simulink model "blocks1"  (R2025a)
settings: Solver=VariableStepAuto  StartTime=0.0  StopTime=10.0  RelTol=1e-3
undefined symbols (not defined in the file or in its folder): physconst
libraries: phaseddetectlib x2, phasedstaplib x1
settings Model: Creator=Admin  LastModifiedBy=Admin

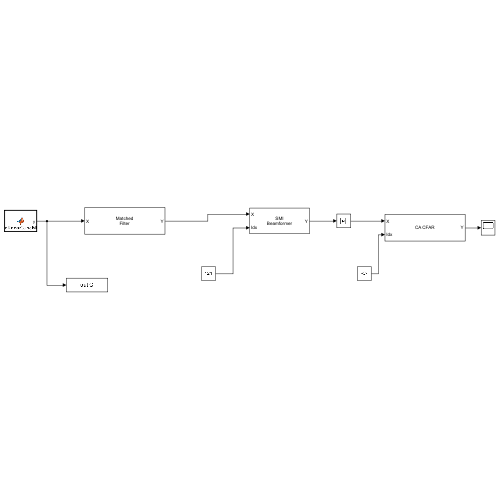
[thumbnail: Simulink's stored preview of the top-level diagram]
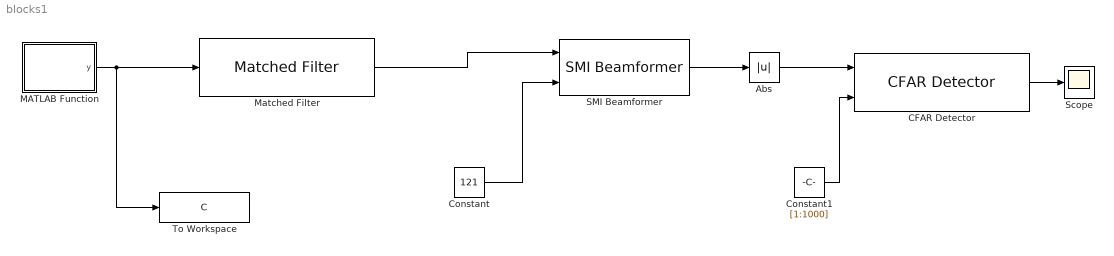
== system blocks1 ==
  Abs : Abs  SaturateOnIntegerOverflow=off
  CFAR Detector : phaseddetectlib/CFAR Detector  Method=CA  Rank=1  NumGuardCells=2  NumTrainingCells=2  ThresholdFactor=Auto  ProbabilityFalseAlarm=0.1  CustomThresholdFactor=1  OutputFormat=CUT result  ThresholdOutputPort=off  NoisePowerOutputPort=off  NumDetectionsSource=Auto  NumDetections=1  SimulateUsing=Interpreted execution
  Constant : Constant  Value=121
  Constant1 : Constant  Value=[1:1000]
  MATLAB Function : MATLAB Function  TreatAsAtomicUnit=on
  Matched Filter : phaseddetectlib/Matched Filter  CoefficientsSource=Property  Coefficients=[ 1; 1 ]  SpectrumWindow=None  CustomSpectrumWindow=@hamming  SpectrumRange=[ 0, 1e5 ]  SampleRateFromInputCheckbox=on  SampleRate=1e6  SidelobeAttenuation=30  Beta=0.5  Nbar=4  GainOutputPort=off  MaximumNumInputSamplesSource=Auto  MaximumNumInputSamples=100  SimulateUsing=Interpreted execution
  SMI Beamformer : phasedstaplib/SMI Beamformer  PropagationSpeed=physconst( 'LightSpeed' )  OperatingFrequency=3e8  PRFSource=Property  PRF=1  DirectionSource=Property  Direction=[ 0; 0 ]  NumPhaseShifterBits=0  DopplerSource=Property  Doppler=0  NumGuardCells=2  NumTrainingCells=2  WeightsOutputPort=off  SimulateUsing=Interpreted execution  SensorArray=phased.URA(Element=phased.IsotropicAntennaElement(),Size=[ 2, 4 ])
  Scope : Scope
      settings: ActiveDisplayYMinimum=-0.30588146868805721  ActiveDisplayYMaximum=1.8509369249247456
  To Workspace : ToWorkspace  VariableName=C  SaveFormat=Structure  SampleTime=-1
      settings: Save2DSignal=2-D array (concatenate along first dimension)
  wires:
  SMI Beamformer/1 -> Abs/1
  Matched Filter/1 -> SMI Beamformer/1
  Constant1/1 -> CFAR Detector/2
  Constant/1 -> SMI Beamformer/2
  Abs/1 -> CFAR Detector/1
  MATLAB Function/1(y) -> To Workspace/1, Matched Filter/1
  CFAR Detector/1 -> Scope/1

== matlab function blocks1/MATLAB Function ==
  data: y output
function y = simulateRadarCubeMF_URA()
%#codegen
% Returns matched-filtered radar data cube [samples x elements x pulses] for URA

% === Parameters ===
nRows = 2;              % URA rows (elevation)
nCols = 4;              % URA cols (azimuth)
nElements = nRows * nCols;
nPulses = 16;
fs = 1e6;
prf = 1000;
pw = 1e-4;
fc = 300e6;
lambda = physconst('LightSpeed') / fc;

% === Waveform ===
waveform = phased.LinearFMWaveform( ...
    'SampleRate', fs, ...
    'PRF', prf, ...
    'PulseWidth', pw);
nSamples = fs / prf;
refPulse = getMatchedFilter(waveform);

% === URA Antenna ===
dy = lambda / 2;
dx = lambda / 2;
antenna = phased.URA('Size', [nRows, nCols], ...
                     'ElementSpacing', [dy, dx]);

% === Radar and Target Components ===
TX = phased.Transmitter('Gain', 20);
TgtModel = phased.RadarTarget;

tgtPos = [10e3 * sqrt(3); 10e3; 0];
tgtVel = [75 * sqrt(3); 75; 0];
PlatformModel = phased.Platform('InitialPosition', tgtPos, ...
                                'Velocity', tgtVel);
ChannelModel = phased.FreeSpace('TwoWayPropagation', true, ...
                                'SampleRate', fs, ...
                                'OperatingFrequency', fc);

txArray = phased.Radiator('Sensor', antenna, ...
                          'OperatingFrequency', fc);
rxArray = phased.Collector('Sensor', antenna, ...
                           'OperatingFrequency', fc);
rxPreamp = phased.ReceiverPreamp('Gain', 10, ...
                                 'NoiseFigure', 5, ...
                                 'SampleRate', fs);

radarPos = [0;0;0];
radarVel = [0;0;0];

% === Preallocate ===
dataCube = complex(zeros(nSamples, nElements, nPulses));

% === Loop over pulses ===
for ii = 1:nPulses
    wf = waveform();
    [tgtPos, tgtVel] = PlatformModel(1/prf);
    [~, tgtAng] = rangeangle(tgtPos, radarPos);

    s0 = TX(wf);
    s1 = txArray(s0, tgtAng);
    s2 = ChannelModel(s1, radarPos, tgtPos, radarVel, tgtVel);
    s3 = TgtModel(s2);
    s4 = rxArray(s3, tgtAng);
    s5 = rxPreamp(s4);

    % === Matched Filter per element ===
    for el = 1:nElements
        dataCube(:, el, ii) = conv(s5(:,el), refPulse, 'same');
    end
end

y = dataCube;  % Return 3D matched-filtered cube
end
